simulink model "closedLoop_toTune"  (R2019a)
settings: Solver=ode14x  StartTime=0.0  StopTime=20  FixedStep=ts  RelTol=1e-3
PreLoadFcn:
  | h = 0.005;
  | k = 0.5;
PostLoadFcn:
  | controlParameters;
undefined symbols (not defined in the file): sigbuilder_block, ts
libraries: simulink x12, controlLibrary x12, mechLibrary x1
CloseFcn:
  | try,close(h1_elec_motor_brushless_dc),end
  | clear h1_elec_motor_brushless_dc
  | 
  | clear simlog_elec_motor_brushless_dc
  | clear logsout_elec_motor_brushless_dc
  | 
  | 
  | clear tout
Description:
  | Position feedback control, with servomotors, of a robot arm. Controllers are discretised.
  | 
  | Copyright 2008-2019 The MathWorks, Inc.
settings Model: DataDictionary=robotDataDictionary.sldd  EnableAccessToBaseWorkspace=off  Creator=MathWorks  LastModifiedBy=falderis
settings ConfigSet: Description=Configuration set for closed loop system
settings SolverCC: ExtrapolationOrder=1  SolverJacobianMethodControl=SparsePerturbation  AutoInsertRateTranBlk=on
settings DataIOCC: SaveFormat=StructureWithTime  SaveOutput=off  ReturnWorkspaceOutputsName=simulationOutput
settings OptimizationCC: BlockReduction=off  OptimizeBlockIOStorage=off  BufferReuse=off  GlobalBufferReuse=off  ExpressionFolding=off  LocalBlockOutputs=off  OptimizeDataStoreBuffers=off  BusAssignmentInplaceUpdate=off
settings DebuggingCC: BusObjectLabelMismatch=none  SFUnexpectedBacktrackingDiag=warning  SFNoUnconditionalDefaultTransitionDiag=warning  SFExecutionAtInitializationDiag=none  ArithmeticOperatorsInVariantConditions=warning
settings HardwareCC: ProdBitPerPointer=32  ProdBitPerSizeT=32  ProdBitPerPtrDiffT=32  ProdLargestAtomicFloat=None  ProdWordSize=32  ProdLongLongMode=on  ProdHWDeviceType=Generic->32-bit x86 compatible
settings ModelReferenceCC: ModelReferenceNumInstancesAllowed=Single  PropagateSignalLabelsOutOfModel=off
settings SFSimCC: SimUseLocalCustomCode=off
settings RTWCC: SystemTargetFile=slrt.tlc  TemplateMakefile=slrt_default_tmf  Description=Simulink Real-Time  RTWVerbose=off  RTWUseLocalCustomCode=off  CodeExecutionProfiling=on  RTWCompilerOptimization=on
settings CodeAppCC: StateflowObjectComments=on
settings SimulinkRealTimeCC: SupportVariableSizeSignals=on  PreserveStateflowLocalDataDimensions=off  RL32LogBufSizeModifier=10000000  xPCConcurrentTasks=on
settings ConfigComp: CovMetricSettings=dw  CovHtmlReporting=on  CovSaveCumulativeToWorkspaceVar=on  CovSaveSingleToWorkspaceVar=on  CovExternalEMLEnable=off  CovSFcnEnable=off
settings SimscapeCC: SimscapeNormalizeSystem=off  SimscapeLogName=mechPlant_simlog  SimscapeLogLimitData=off
settings ConfigurationSet: Description=SimMechanics 2G
settings ExplorerConfigSet: InternalSimMechanicsExplorerSettings="<ExplorerConfiguration><canonicalview>planar_xy</canonicalview><AnimationSetting><BasePlaybackSpeed>1.0</BasePlaybackSpeed><PlaybackSpeedFactor>0.5</PlaybackSpeedFactor></AnimationSetting><TilePanel><TileInfo><Tiles Columns=\"1\" Count=\"1\" Rows=\"1\"><Column Weight=\"1\"/><Row Weight=\"1\"/><Tile Height=\"1\" Width=\"1\" X=\"0\" Y=\"0\"/></Tiles></TileInfo><SceneInfo><SceneViewer><BGColor><R>1</R><G>1</G><B>1</B></BGColor><Camera><DoPerspective>off</DoPerspective><Position><X>0.403135839827215292</X><Y>0.401665542364257</Y><Z>0.341712609240549303</Z></Position><Center><X>0.0802051411090622807</X><Y>0.078734843646070099</Y><Z>0.0187819105223669576</Z></Center><Up><X>-0.408248290463863073</X><Y>0.816496580927726145</Y><Z>-0.408248290463863073</Z></Up><ViewLimDist>1</ViewLimDist><YLim>0.277558730438193679</YLim><XLim>0.533545538821605492</XLim></Camera></SceneViewer></SceneInfo></TilePanel><MechEditorPanel><Cameras/><GfxPanelCameraMap/><VideoCreator><PlaybackSpeedRatio>1.0</PlaybackSpeedRatio><FrameRate>30</FrameRate><VideoFormat>Motion JPEG AVI</VideoFormat><FrameSize>auto</FrameSize></VideoCreator></MechEditorPanel></ExplorerConfiguration>"

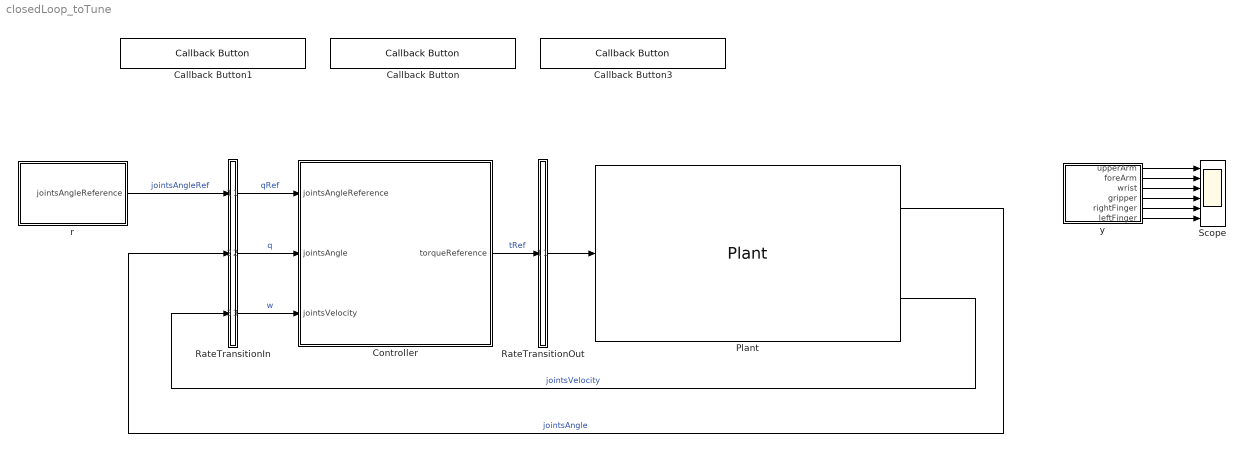
== system closedLoop_toTune ==
  Callback Button : CallbackButton  ButtonText=Open Control System Tuner
      settings: ClickFcn=|
      | h = 0.005;
      | k = 0.5;
      | controlParameters;
      | controlSystemTuner('ControlSystemTunerSession.mat')
  Callback Button1 : CallbackButton  ButtonText=Untuned Controllers
      settings: ClickFcn=|
      | h = 0.005;
      | k = 0.5;
      | controlParameters;
  Callback Button3 : CallbackButton  ButtonText=Aggressive Controller
      settings: ClickFcn=|
      | h = 1;
      | k = 1;
      | controlParameters;
  Controller : Subsystem
      mask Display: image('controller.png')
  Plant : mechLibrary/Plant  SystemSampleTime=-1
  RateTransitionIn : Subsystem
  RateTransitionOut : Subsystem
  Scope : Scope  NumInputPorts=6
  r : Subsystem
      mask Display: disp('input')
  y : Subsystem
      mask Display: disp('output')
  wires:
  Controller/1(torqueReference) -> RateTransitionOut/1(tRefIn)  "tRef"
  RateTransitionIn/1(qRef) -> Controller/1(jointsAngleReference)  "qRef"
  Plant/2 -> RateTransitionIn/3(wIn)  "jointsVelocity"
  RateTransitionOut/1(tRef) -> Plant/1
  RateTransitionIn/3(w) -> Controller/3(jointsVelocity)  "w"
  Plant/1 -> RateTransitionIn/2(qIn)  "jointsAngle"
  RateTransitionIn/2(q) -> Controller/2(jointsAngle)  "q"
  r/1(jointsAngleReference) -> RateTransitionIn/1(qRefIn)  "jointsAngleRef"
  y/1(upperArm) -> Scope/1
  y/2(foreArm) -> Scope/2
  y/3(wrist) -> Scope/3
  y/4(gripper) -> Scope/4
  y/5(rightFinger) -> Scope/5
  y/6(leftFinger) -> Scope/6

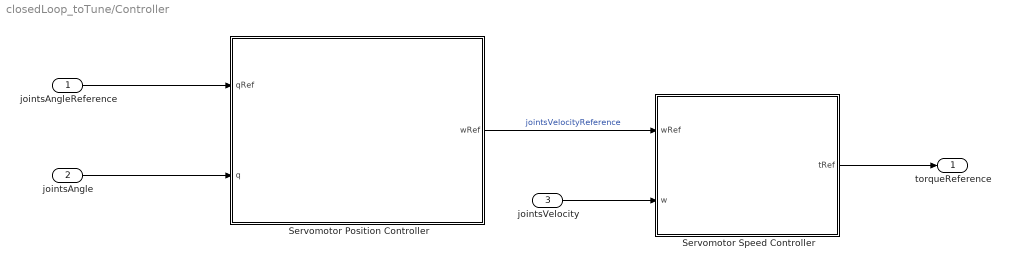
== system closedLoop_toTune/Controller ==
  jointsAngleReference : Inport  OutDataTypeStr=Bus: jointMotionBus  Unit=deg  SampleTime=ts
  jointsAngle : Inport  Port=2  OutDataTypeStr=Bus: jointMotionBus  Unit=deg  SampleTime=ts
  jointsVelocity : Inport  Port=3  OutDataTypeStr=Bus: jointVelBus  Unit=deg/s  SampleTime=ts
  Servomotor Position Controller : Subsystem  VariantControl=SV
      mask Display: image('pid.png');
  Servomotor Speed Controller : Subsystem
      mask Display: image('pi2.png');
  torqueReference : Outport  OutDataTypeStr=Bus: jointTorqueBus  Unit=N*m  SampleTime=ts
  wires:
  jointsAngle/1 -> Servomotor Position Controller/2(q)
  jointsAngleReference/1 -> Servomotor Position Controller/1(qRef)
  Servomotor Speed Controller/1(tRef) -> torqueReference/1
  Servomotor Position Controller/1(wRef) -> Servomotor Speed Controller/1(wRef)  "jointsVelocityReference"
  jointsVelocity/1 -> Servomotor Speed Controller/2(w)

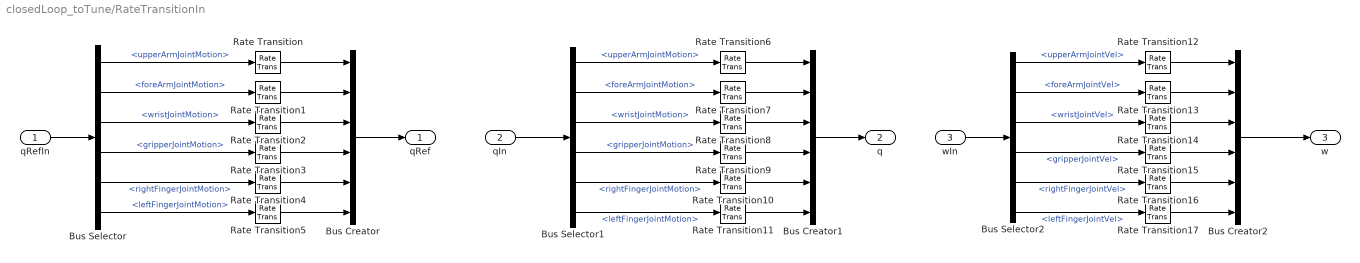
== system closedLoop_toTune/RateTransitionIn ==
  qRefIn : Inport  OutDataTypeStr=Bus: jointMotionBus  Unit=deg
  qIn : Inport  Port=2  OutDataTypeStr=Bus: jointMotionBus  Unit=deg
  wIn : Inport  Port=3  OutDataTypeStr=Bus: jointVelBus
  Bus Creator : BusCreator  Inputs=6  OutDataTypeStr=Bus: jointMotionBus
      settings: InheritFromInputs=off
  Bus Creator1 : BusCreator  Inputs=6  OutDataTypeStr=Bus: jointMotionBus
      settings: InheritFromInputs=off
  Bus Creator2 : BusCreator  Inputs=6  OutDataTypeStr=Bus: jointVelBus
      settings: InheritFromInputs=off
  Bus Selector : BusSelector  OutputSignals=upperArmJointMotion,foreArmJointMotion,wristJointMotion,gripperJointMotion,rightFingerJointMotion,leftFingerJointMotion
  Bus Selector1 : BusSelector  OutputSignals=upperArmJointMotion,foreArmJointMotion,wristJointMotion,gripperJointMotion,rightFingerJointMotion,leftFingerJointMotion
  Bus Selector2 : BusSelector  OutputSignals=upperArmJointVel,foreArmJointVel,wristJointVel,gripperJointVel,rightFingerJointVel,leftFingerJointVel
  Rate Transition{,1..17} (18 alike) : RateTransition  OutPortSampleTime=ts
  qRef : Outport  OutDataTypeStr=Bus: jointMotionBus
  q : Outport  Port=2  OutDataTypeStr=Bus: jointMotionBus
  w : Outport  Port=3  OutDataTypeStr=Bus: jointVelBus
  wires:
  Bus Selector1/6 -> Rate Transition11/1  "<leftFingerJointMotion>"
  Bus Selector1/3 -> Rate Transition8/1  "<wristJointMotion>"
  qIn/1 -> Bus Selector1/1
  Bus Selector1/1 -> Rate Transition6/1  "<upperArmJointMotion>"
  Bus Selector1/5 -> Rate Transition10/1  "<rightFingerJointMotion>"
  Bus Selector/6 -> Rate Transition5/1  "<leftFingerJointMotion>"
  Bus Selector1/4 -> Rate Transition9/1  "<gripperJointMotion>"
  Bus Selector/2 -> Rate Transition1/1  "<foreArmJointMotion>"
  Bus Selector1/2 -> Rate Transition7/1  "<foreArmJointMotion>"
  Bus Selector/3 -> Rate Transition2/1  "<wristJointMotion>"
  Bus Selector/4 -> Rate Transition3/1  "<gripperJointMotion>"
  Bus Selector/1 -> Rate Transition/1  "<upperArmJointMotion>"
  qRefIn/1 -> Bus Selector/1
  Bus Selector/5 -> Rate Transition4/1  "<rightFingerJointMotion>"
  Bus Selector2/5 -> Rate Transition16/1  "<rightFingerJointVel>"
  Bus Selector2/4 -> Rate Transition15/1  "<gripperJointVel>"
  Bus Selector2/3 -> Rate Transition14/1  "<wristJointVel>"
  wIn/1 -> Bus Selector2/1
  Bus Selector2/1 -> Rate Transition12/1  "<upperArmJointVel>"
  Bus Selector2/2 -> Rate Transition13/1  "<foreArmJointVel>"
  Bus Selector2/6 -> Rate Transition17/1  "<leftFingerJointVel>"
  Rate Transition/1 -> Bus Creator/1
  Rate Transition1/1 -> Bus Creator/2
  Rate Transition2/1 -> Bus Creator/3
  Rate Transition3/1 -> Bus Creator/4
  Rate Transition4/1 -> Bus Creator/5
  Rate Transition5/1 -> Bus Creator/6
  Bus Creator/1 -> qRef/1
  Rate Transition7/1 -> Bus Creator1/2
  Rate Transition11/1 -> Bus Creator1/6
  Bus Creator1/1 -> q/1
  Rate Transition9/1 -> Bus Creator1/4
  Rate Transition6/1 -> Bus Creator1/1
  Rate Transition8/1 -> Bus Creator1/3
  Rate Transition10/1 -> Bus Creator1/5
  Rate Transition12/1 -> Bus Creator2/1
  Rate Transition13/1 -> Bus Creator2/2
  Rate Transition14/1 -> Bus Creator2/3
  Rate Transition15/1 -> Bus Creator2/4
  Rate Transition16/1 -> Bus Creator2/5
  Rate Transition17/1 -> Bus Creator2/6
  Bus Creator2/1 -> w/1

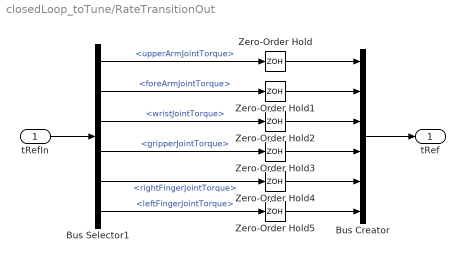
== system closedLoop_toTune/RateTransitionOut ==
  tRefIn : Inport  OutDataTypeStr=Bus: jointTorqueBus  Unit=N*m
  Bus Creator : BusCreator  Inputs=6  OutDataTypeStr=Bus: jointTorqueBus
      settings: InheritFromInputs=off
  Bus Selector1 : BusSelector  OutputSignals=upperArmJointTorque,foreArmJointTorque,wristJointTorque,gripperJointTorque,rightFingerJointTorque,leftFingerJointTorque
  Zero-Order Hold{,1..5} (6 alike) : ZeroOrderHold  SampleTime=-1
  tRef : Outport  OutDataTypeStr=Bus: jointTorqueBus  SampleTime=0
  wires:
  Bus Selector1/3 -> Zero-Order Hold2/1  "<wristJointTorque>"
  tRefIn/1 -> Bus Selector1/1
  Bus Selector1/2 -> Zero-Order Hold1/1  "<foreArmJointTorque>"
  Bus Selector1/5 -> Zero-Order Hold4/1  "<rightFingerJointTorque>"
  Bus Selector1/4 -> Zero-Order Hold3/1  "<gripperJointTorque>"
  Bus Selector1/1 -> Zero-Order Hold/1  "<upperArmJointTorque>"
  Bus Selector1/6 -> Zero-Order Hold5/1  "<leftFingerJointTorque>"
  Zero-Order Hold5/1 -> Bus Creator/6
  Zero-Order Hold4/1 -> Bus Creator/5
  Zero-Order Hold1/1 -> Bus Creator/2
  Zero-Order Hold/1 -> Bus Creator/1
  Zero-Order Hold2/1 -> Bus Creator/3
  Zero-Order Hold3/1 -> Bus Creator/4
  Bus Creator/1 -> tRef/1

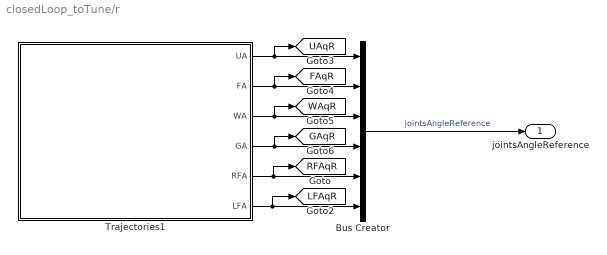
== system closedLoop_toTune/r ==
  Bus Creator : BusCreator  Inputs=6  OutDataTypeStr=Bus: jointMotionBus
      settings: InheritFromInputs=off
  Trajectories1 : Subsystem  Tag=STV Subsys  LoadFcn=sigbuilder_block('load');  StartFcn=sigbuilder_block('start');  StopFcn=sigbuilder_block('stop');  ClipboardFcn=sigbuilder_block('clipboard');  mask(Sigbuilder block){tuvar=[0:10]}
      mask help: Simulink:masks:SigbuilderBlock_MD
      mask init:
      | if ~strcmp(get_param(bdroot(gcbh),'SimulationStatus'),'stopped') tuvar = sigbuilder_block('maskInit'); end
      settings: CopyFcn=sigbuilder_block('copy');  DeleteFcn=sigbuilder_block('delete');  ModelCloseFcn=sigbuilder_block('modelClose');  PreSaveFcn=sigbuilder_block('preSave');  PauseFcn=sigbuilder_block('pause');  ContinueFcn=sigbuilder_block('continue');  NameChangeFcn=sigbuilder_block('namechange');  OpenFcn=sigbuilder_block('open',[0 30 1440 722.25 ]);  CloseFcn=sigbuilder_block('close');
      mask Display: plot(0, 0, 100, 100,[2, 2, 32, 32, 2], [68, 8, 8, 68, 68],[32, 2], [38, 38], [32, 19, 2],[53, 60, 44], [32, 17, 17, 2],[16, 16, 31, 31]);txt = getActiveGroup(gcbh);text(2, 100, txt,'verticalAlignment', 'top');
  jointsAngleReference : Outport
  tag scope: FAqR=global, GAqR=global, LFAqR=global, RFAqR=global, UAqR=global, WAqR=global
  wires:
  Trajectories1/6(LFA) -> Bus Creator/6, [LFAqR]
  Trajectories1/2(FA) -> Bus Creator/2, [FAqR]
  Trajectories1/5(RFA) -> Bus Creator/5, [RFAqR]
  Trajectories1/1(UA) -> [UAqR], Bus Creator/1
  Trajectories1/4(GA) -> [GAqR], Bus Creator/4
  Trajectories1/3(WA) -> [WAqR], Bus Creator/3
  Bus Creator/1 -> jointsAngleReference/1  "jointsAngleReference"

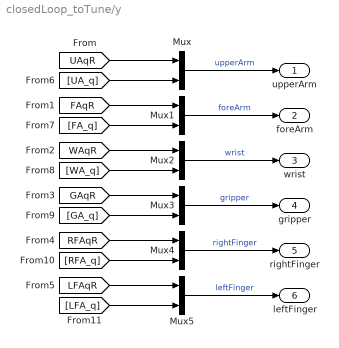
== system closedLoop_toTune/y ==
  Mux{,1..5} (6 alike) : Mux  Inputs=2
  upperArm : Outport
  foreArm : Outport  Port=2
  wrist : Outport  Port=3
  gripper : Outport  Port=4
  rightFinger : Outport  Port=5
  leftFinger : Outport  Port=6
  wires:
  Mux5/1 -> leftFinger/1  "leftFinger"
  [UA_q] -> Mux/2
  [RFA_q] -> Mux4/2
  [RFAqR] -> Mux4/1
  [UAqR] -> Mux/1
  [FAqR] -> Mux1/1
  [WAqR] -> Mux2/1
  [WA_q] -> Mux2/2
  [FA_q] -> Mux1/2
  [LFAqR] -> Mux5/1
  [LFA_q] -> Mux5/2
  [GAqR] -> Mux3/1
  [GA_q] -> Mux3/2
  Mux/1 -> upperArm/1  "upperArm"
  Mux1/1 -> foreArm/1  "foreArm"
  Mux2/1 -> wrist/1  "wrist"
  Mux4/1 -> rightFinger/1  "rightFinger"
  Mux3/1 -> gripper/1  "gripper"

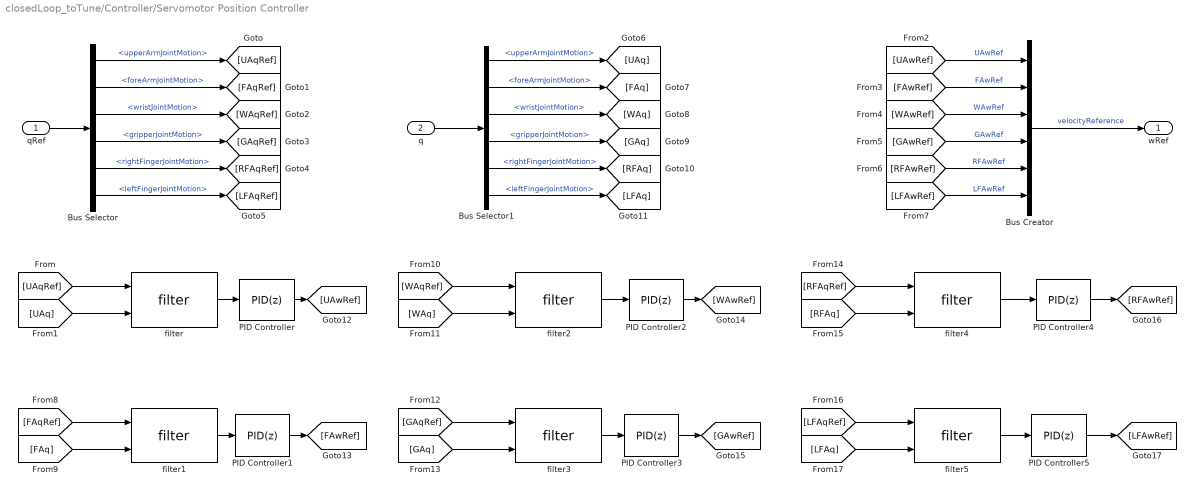
== system closedLoop_toTune/Controller/Servomotor Position Controller ==
  qRef : Inport  OutDataTypeStr=Bus: jointMotionBus  Unit=deg
  q : Inport  Port=2  OutDataTypeStr=Bus: jointMotionBus  Unit=deg
  Bus Creator : BusCreator  Inputs=6  OutDataTypeStr=Bus: jointVelBus
      settings: InheritFromInputs=off
  Bus Selector : BusSelector  OutputSignals=upperArmJointMotion,foreArmJointMotion,wristJointMotion,gripperJointMotion,rightFingerJointMotion,leftFingerJointMotion
  Bus Selector1 : BusSelector  OutputSignals=upperArmJointMotion,foreArmJointMotion,wristJointMotion,gripperJointMotion,rightFingerJointMotion,leftFingerJointMotion
  PID Controller : simulink/Continuous/PID Controller  Controller=PID  Form=Parallel  TimeDomain=Discrete-time  SampleTime=ts  IntegratorMethod=Forward Euler  FilterMethod=Forward Euler  ControllerParametersSource=internal  P=0.58  I=4.83  D=0.0027  UseFilter=on  N=0.95  TunerSelectOption=Transfer Function Based (PID Tuner App)  InitialConditionSource=internal  InitialConditionForIntegrator=0  InitialConditionForFilter=0  DifferentiatorICPrevScaledInput=0  ExternalReset=none  TrackingMode=off  Kt=1  LimitOutput=off  UpperSaturationLimit=inf  LowerSaturationLimit=-inf  LinearizeAsGain=on  AntiWindupMode=none  Kb=1  POutMin=[]  POutMax=[]  IOutMin=[]  IOutMax=[]  DOutMin=[]  DOutMax=[]  NOutMin=[]  NOutMax=[]  SumOutMin=[]  SumOutMax=[]  SaturationOutMin=[]  SaturationOutMax=[]  PParamMin=[]  PParamMax=[]  IParamMin=[]  IParamMax=[]  DParamMin=[]  DParamMax=[]  NParamMin=[]  NParamMax=[]  KbParamMin=[]  KbParamMax=[]  KtParamMin=[]  KtParamMax=[]  KbOutMin=[]  KbOutMax=[]  KtOutMin=[]  KtOutMax=[]  IntegratorOutMin=[]  IntegratorOutMax=[]  FilterOutMin=[]  FilterOutMax=[]  SumI1OutMin=[]  SumI1OutMax=[]  SumI2OutMin=[]  SumI2OutMax=[]  SumI3OutMin=[]  SumI3OutMax=[]  SumI4OutMin=[]  SumI4OutMax=[]  SumDOutMin=[]  SumDOutMax=[]  DifferentiatorOutMin=[]  DifferentiatorOutMax=[]  FilterDiffOutCoefMin=[]  FilterDiffOutCoefMax=[]  ReciprocalOutMin=[]  ReciprocalOutMax=[]  SumDenOutMin=[]  SumDenOutMax=[]  SumNumOutMin=[]  SumNumOutMax=[]  DivideOutMin=[]  DivideOutMax=[]  IntegratorContinuousStateAttributes=''  IntegratorStateMustResolveToSignalObject=off  IntegratorRTWStateStorageClass=Auto  FilterContinuousStateAttributes=''  FilterStateMustResolveToSignalObject=off  FilterRTWStateStorageClass=Auto  ParallelPVariant=InternalParameters  IdealPVariant=Disabled  IVariant=InternalParameters  DVariant=InternalParameters  IntegratorVariant=Discrete  SatVariant=Disabled  AWVariant=Passthrough  PCopyVariant=Disabled  TRVariant=Disabled  FdbkBlocksVariant=Forward  IdealPFdbkVariant=Disabled  SatFdbkVariant=Disabled  DerivativeFilterVariant=ForwardEulerFilter  NVariant=InternalParameters  NCopyVariant=Disabled  FilterICVariant=InternalICsFilter  IntegratorICVariant=InternalICs  ExternalResetVariant=Disabled  TRSumVariant=Passthrough  SumFdbkVariant=Disabled  SumVariant=Sum_PID
  PID Controller1 : simulink/Continuous/PID Controller  Controller=PID  Form=Parallel  TimeDomain=Discrete-time  SampleTime=ts  IntegratorMethod=Forward Euler  FilterMethod=Forward Euler  ControllerParametersSource=internal  P=0.11915  I=0.918  D=0.00315  UseFilter=on  N=1.15  TunerSelectOption=Transfer Function Based (PID Tuner App)  InitialConditionSource=internal  InitialConditionForIntegrator=0  InitialConditionForFilter=0  DifferentiatorICPrevScaledInput=0  ExternalReset=none  TrackingMode=off  Kt=1  LimitOutput=off  UpperSaturationLimit=inf  LowerSaturationLimit=-inf  LinearizeAsGain=on  AntiWindupMode=none  Kb=1  POutMin=[]  POutMax=[]  IOutMin=[]  IOutMax=[]  DOutMin=[]  DOutMax=[]  NOutMin=[]  NOutMax=[]  SumOutMin=[]  SumOutMax=[]  SaturationOutMin=[]  SaturationOutMax=[]  PParamMin=[]  PParamMax=[]  IParamMin=[]  IParamMax=[]  DParamMin=[]  DParamMax=[]  NParamMin=[]  NParamMax=[]  KbParamMin=[]  KbParamMax=[]  KtParamMin=[]  KtParamMax=[]  KbOutMin=[]  KbOutMax=[]  KtOutMin=[]  KtOutMax=[]  IntegratorOutMin=[]  IntegratorOutMax=[]  FilterOutMin=[]  FilterOutMax=[]  SumI1OutMin=[]  SumI1OutMax=[]  SumI2OutMin=[]  SumI2OutMax=[]  SumI3OutMin=[]  SumI3OutMax=[]  SumI4OutMin=[]  SumI4OutMax=[]  SumDOutMin=[]  SumDOutMax=[]  DifferentiatorOutMin=[]  DifferentiatorOutMax=[]  FilterDiffOutCoefMin=[]  FilterDiffOutCoefMax=[]  ReciprocalOutMin=[]  ReciprocalOutMax=[]  SumDenOutMin=[]  SumDenOutMax=[]  SumNumOutMin=[]  SumNumOutMax=[]  DivideOutMin=[]  DivideOutMax=[]  IntegratorContinuousStateAttributes=''  IntegratorStateMustResolveToSignalObject=off  IntegratorRTWStateStorageClass=Auto  FilterContinuousStateAttributes=''  FilterStateMustResolveToSignalObject=off  FilterRTWStateStorageClass=Auto  ParallelPVariant=InternalParameters  IdealPVariant=Disabled  IVariant=InternalParameters  DVariant=InternalParameters  IntegratorVariant=Discrete  SatVariant=Disabled  AWVariant=Passthrough  PCopyVariant=Disabled  TRVariant=Disabled  FdbkBlocksVariant=Forward  IdealPFdbkVariant=Disabled  SatFdbkVariant=Disabled  DerivativeFilterVariant=ForwardEulerFilter  NVariant=InternalParameters  NCopyVariant=Disabled  FilterICVariant=InternalICsFilter  IntegratorICVariant=InternalICs  ExternalResetVariant=Disabled  TRSumVariant=Passthrough  SumFdbkVariant=Disabled  SumVariant=Sum_PID
  PID Controller2 : simulink/Continuous/PID Controller  Controller=PID  Form=Parallel  TimeDomain=Discrete-time  SampleTime=ts  IntegratorMethod=Forward Euler  FilterMethod=Forward Euler  ControllerParametersSource=internal  P=0.468  I=3.6488  D=0.0031  UseFilter=on  N=3.7035  TunerSelectOption=Transfer Function Based (PID Tuner App)  InitialConditionSource=internal  InitialConditionForIntegrator=0  InitialConditionForFilter=0  DifferentiatorICPrevScaledInput=0  ExternalReset=none  TrackingMode=off  Kt=1  LimitOutput=off  UpperSaturationLimit=inf  LowerSaturationLimit=-inf  LinearizeAsGain=on  AntiWindupMode=none  Kb=1  POutMin=[]  POutMax=[]  IOutMin=[]  IOutMax=[]  DOutMin=[]  DOutMax=[]  NOutMin=[]  NOutMax=[]  SumOutMin=[]  SumOutMax=[]  SaturationOutMin=[]  SaturationOutMax=[]  PParamMin=[]  PParamMax=[]  IParamMin=[]  IParamMax=[]  DParamMin=[]  DParamMax=[]  NParamMin=[]  NParamMax=[]  KbParamMin=[]  KbParamMax=[]  KtParamMin=[]  KtParamMax=[]  KbOutMin=[]  KbOutMax=[]  KtOutMin=[]  KtOutMax=[]  IntegratorOutMin=[]  IntegratorOutMax=[]  FilterOutMin=[]  FilterOutMax=[]  SumI1OutMin=[]  SumI1OutMax=[]  SumI2OutMin=[]  SumI2OutMax=[]  SumI3OutMin=[]  SumI3OutMax=[]  SumI4OutMin=[]  SumI4OutMax=[]  SumDOutMin=[]  SumDOutMax=[]  DifferentiatorOutMin=[]  DifferentiatorOutMax=[]  FilterDiffOutCoefMin=[]  FilterDiffOutCoefMax=[]  ReciprocalOutMin=[]  ReciprocalOutMax=[]  SumDenOutMin=[]  SumDenOutMax=[]  SumNumOutMin=[]  SumNumOutMax=[]  DivideOutMin=[]  DivideOutMax=[]  IntegratorContinuousStateAttributes=''  IntegratorStateMustResolveToSignalObject=off  IntegratorRTWStateStorageClass=Auto  FilterContinuousStateAttributes=''  FilterStateMustResolveToSignalObject=off  FilterRTWStateStorageClass=Auto  ParallelPVariant=InternalParameters  IdealPVariant=Disabled  IVariant=InternalParameters  DVariant=InternalParameters  IntegratorVariant=Discrete  SatVariant=Disabled  AWVariant=Passthrough  PCopyVariant=Disabled  TRVariant=Disabled  FdbkBlocksVariant=Forward  IdealPFdbkVariant=Disabled  SatFdbkVariant=Disabled  DerivativeFilterVariant=ForwardEulerFilter  NVariant=InternalParameters  NCopyVariant=Disabled  FilterICVariant=InternalICsFilter  IntegratorICVariant=InternalICs  ExternalResetVariant=Disabled  TRSumVariant=Passthrough  SumFdbkVariant=Disabled  SumVariant=Sum_PID
  PID Controller3 : simulink/Continuous/PID Controller  Controller=PID  Form=Parallel  TimeDomain=Discrete-time  SampleTime=ts  IntegratorMethod=Forward Euler  FilterMethod=Forward Euler  ControllerParametersSource=internal  P=0.30195  I=0.20875  D=0.00335  UseFilter=on  N=3.677  TunerSelectOption=Transfer Function Based (PID Tuner App)  InitialConditionSource=internal  InitialConditionForIntegrator=0  InitialConditionForFilter=0  DifferentiatorICPrevScaledInput=0  ExternalReset=none  TrackingMode=off  Kt=1  LimitOutput=off  UpperSaturationLimit=inf  LowerSaturationLimit=-inf  LinearizeAsGain=on  AntiWindupMode=none  Kb=1  POutMin=[]  POutMax=[]  IOutMin=[]  IOutMax=[]  DOutMin=[]  DOutMax=[]  NOutMin=[]  NOutMax=[]  SumOutMin=[]  SumOutMax=[]  SaturationOutMin=[]  SaturationOutMax=[]  PParamMin=[]  PParamMax=[]  IParamMin=[]  IParamMax=[]  DParamMin=[]  DParamMax=[]  NParamMin=[]  NParamMax=[]  KbParamMin=[]  KbParamMax=[]  KtParamMin=[]  KtParamMax=[]  KbOutMin=[]  KbOutMax=[]  KtOutMin=[]  KtOutMax=[]  IntegratorOutMin=[]  IntegratorOutMax=[]  FilterOutMin=[]  FilterOutMax=[]  SumI1OutMin=[]  SumI1OutMax=[]  SumI2OutMin=[]  SumI2OutMax=[]  SumI3OutMin=[]  SumI3OutMax=[]  SumI4OutMin=[]  SumI4OutMax=[]  SumDOutMin=[]  SumDOutMax=[]  DifferentiatorOutMin=[]  DifferentiatorOutMax=[]  FilterDiffOutCoefMin=[]  FilterDiffOutCoefMax=[]  ReciprocalOutMin=[]  ReciprocalOutMax=[]  SumDenOutMin=[]  SumDenOutMax=[]  SumNumOutMin=[]  SumNumOutMax=[]  DivideOutMin=[]  DivideOutMax=[]  IntegratorContinuousStateAttributes=''  IntegratorStateMustResolveToSignalObject=off  IntegratorRTWStateStorageClass=Auto  FilterContinuousStateAttributes=''  FilterStateMustResolveToSignalObject=off  FilterRTWStateStorageClass=Auto  ParallelPVariant=InternalParameters  IdealPVariant=Disabled  IVariant=InternalParameters  DVariant=InternalParameters  IntegratorVariant=Discrete  SatVariant=Disabled  AWVariant=Passthrough  PCopyVariant=Disabled  TRVariant=Disabled  FdbkBlocksVariant=Forward  IdealPFdbkVariant=Disabled  SatFdbkVariant=Disabled  DerivativeFilterVariant=ForwardEulerFilter  NVariant=InternalParameters  NCopyVariant=Disabled  FilterICVariant=InternalICsFilter  IntegratorICVariant=InternalICs  ExternalResetVariant=Disabled  TRSumVariant=Passthrough  SumFdbkVariant=Disabled  SumVariant=Sum_PID
  PID Controller4 : simulink/Continuous/PID Controller  Controller=PID  Form=Parallel  TimeDomain=Discrete-time  SampleTime=ts  IntegratorMethod=Forward Euler  FilterMethod=Forward Euler  ControllerParametersSource=internal  P=0.425  I=3.52  D=0.0036  UseFilter=on  N=1.2175  TunerSelectOption=Transfer Function Based (PID Tuner App)  InitialConditionSource=internal  InitialConditionForIntegrator=0  InitialConditionForFilter=0  DifferentiatorICPrevScaledInput=0  ExternalReset=none  TrackingMode=off  Kt=1  LimitOutput=off  UpperSaturationLimit=inf  LowerSaturationLimit=-inf  LinearizeAsGain=on  AntiWindupMode=none  Kb=1  POutMin=[]  POutMax=[]  IOutMin=[]  IOutMax=[]  DOutMin=[]  DOutMax=[]  NOutMin=[]  NOutMax=[]  SumOutMin=[]  SumOutMax=[]  SaturationOutMin=[]  SaturationOutMax=[]  PParamMin=[]  PParamMax=[]  IParamMin=[]  IParamMax=[]  DParamMin=[]  DParamMax=[]  NParamMin=[]  NParamMax=[]  KbParamMin=[]  KbParamMax=[]  KtParamMin=[]  KtParamMax=[]  KbOutMin=[]  KbOutMax=[]  KtOutMin=[]  KtOutMax=[]  IntegratorOutMin=[]  IntegratorOutMax=[]  FilterOutMin=[]  FilterOutMax=[]  SumI1OutMin=[]  SumI1OutMax=[]  SumI2OutMin=[]  SumI2OutMax=[]  SumI3OutMin=[]  SumI3OutMax=[]  SumI4OutMin=[]  SumI4OutMax=[]  SumDOutMin=[]  SumDOutMax=[]  DifferentiatorOutMin=[]  DifferentiatorOutMax=[]  FilterDiffOutCoefMin=[]  FilterDiffOutCoefMax=[]  ReciprocalOutMin=[]  ReciprocalOutMax=[]  SumDenOutMin=[]  SumDenOutMax=[]  SumNumOutMin=[]  SumNumOutMax=[]  DivideOutMin=[]  DivideOutMax=[]  IntegratorContinuousStateAttributes=''  IntegratorStateMustResolveToSignalObject=off  IntegratorRTWStateStorageClass=Auto  FilterContinuousStateAttributes=''  FilterStateMustResolveToSignalObject=off  FilterRTWStateStorageClass=Auto  ParallelPVariant=InternalParameters  IdealPVariant=Disabled  IVariant=InternalParameters  DVariant=InternalParameters  IntegratorVariant=Discrete  SatVariant=Disabled  AWVariant=Passthrough  PCopyVariant=Disabled  TRVariant=Disabled  FdbkBlocksVariant=Forward  IdealPFdbkVariant=Disabled  SatFdbkVariant=Disabled  DerivativeFilterVariant=ForwardEulerFilter  NVariant=InternalParameters  NCopyVariant=Disabled  FilterICVariant=InternalICsFilter  IntegratorICVariant=InternalICs  ExternalResetVariant=Disabled  TRSumVariant=Passthrough  SumFdbkVariant=Disabled  SumVariant=Sum_PID
  PID Controller5 : simulink/Continuous/PID Controller  Controller=PID  Form=Parallel  TimeDomain=Discrete-time  SampleTime=ts  IntegratorMethod=Forward Euler  FilterMethod=Forward Euler  ControllerParametersSource=internal  P=0.58  I=4.83  D=0.0027  UseFilter=on  N=0.95  TunerSelectOption=Transfer Function Based (PID Tuner App)  InitialConditionSource=internal  InitialConditionForIntegrator=0  InitialConditionForFilter=0  DifferentiatorICPrevScaledInput=0  ExternalReset=none  TrackingMode=off  Kt=1  LimitOutput=off  UpperSaturationLimit=inf  LowerSaturationLimit=-inf  LinearizeAsGain=on  AntiWindupMode=none  Kb=1  POutMin=[]  POutMax=[]  IOutMin=[]  IOutMax=[]  DOutMin=[]  DOutMax=[]  NOutMin=[]  NOutMax=[]  SumOutMin=[]  SumOutMax=[]  SaturationOutMin=[]  SaturationOutMax=[]  PParamMin=[]  PParamMax=[]  IParamMin=[]  IParamMax=[]  DParamMin=[]  DParamMax=[]  NParamMin=[]  NParamMax=[]  KbParamMin=[]  KbParamMax=[]  KtParamMin=[]  KtParamMax=[]  KbOutMin=[]  KbOutMax=[]  KtOutMin=[]  KtOutMax=[]  IntegratorOutMin=[]  IntegratorOutMax=[]  FilterOutMin=[]  FilterOutMax=[]  SumI1OutMin=[]  SumI1OutMax=[]  SumI2OutMin=[]  SumI2OutMax=[]  SumI3OutMin=[]  SumI3OutMax=[]  SumI4OutMin=[]  SumI4OutMax=[]  SumDOutMin=[]  SumDOutMax=[]  DifferentiatorOutMin=[]  DifferentiatorOutMax=[]  FilterDiffOutCoefMin=[]  FilterDiffOutCoefMax=[]  ReciprocalOutMin=[]  ReciprocalOutMax=[]  SumDenOutMin=[]  SumDenOutMax=[]  SumNumOutMin=[]  SumNumOutMax=[]  DivideOutMin=[]  DivideOutMax=[]  IntegratorContinuousStateAttributes=''  IntegratorStateMustResolveToSignalObject=off  IntegratorRTWStateStorageClass=Auto  FilterContinuousStateAttributes=''  FilterStateMustResolveToSignalObject=off  FilterRTWStateStorageClass=Auto  ParallelPVariant=InternalParameters  IdealPVariant=Disabled  IVariant=InternalParameters  DVariant=InternalParameters  IntegratorVariant=Discrete  SatVariant=Disabled  AWVariant=Passthrough  PCopyVariant=Disabled  TRVariant=Disabled  FdbkBlocksVariant=Forward  IdealPFdbkVariant=Disabled  SatFdbkVariant=Disabled  DerivativeFilterVariant=ForwardEulerFilter  NVariant=InternalParameters  NCopyVariant=Disabled  FilterICVariant=InternalICsFilter  IntegratorICVariant=InternalICs  ExternalResetVariant=Disabled  TRSumVariant=Passthrough  SumFdbkVariant=Disabled  SumVariant=Sum_PID
  filter{,1..5} (6 alike) : controlLibrary/filter  tc=1e-2  sampleTime=ts
  wRef : Outport  OutDataTypeStr=Bus: jointVelBus  Unit=deg/s
  wires:
  qRef/1 -> Bus Selector/1
  q/1 -> Bus Selector1/1
  Bus Selector/1 -> [UAqRef]  "<upperArmJointMotion>"
  Bus Selector/2 -> [FAqRef]  "<foreArmJointMotion>"
  Bus Selector/3 -> [WAqRef]  "<wristJointMotion>"
  Bus Selector/4 -> [GAqRef]  "<gripperJointMotion>"
  Bus Selector/5 -> [RFAqRef]  "<rightFingerJointMotion>"
  Bus Selector/6 -> [LFAqRef]  "<leftFingerJointMotion>"
  Bus Selector1/1 -> [UAq]  "<upperArmJointMotion>"
  Bus Selector1/3 -> [WAq]  "<wristJointMotion>"
  Bus Selector1/2 -> [FAq]  "<foreArmJointMotion>"
  Bus Selector1/5 -> [RFAq]  "<rightFingerJointMotion>"
  Bus Selector1/4 -> [GAq]  "<gripperJointMotion>"
  Bus Selector1/6 -> [LFAq]  "<leftFingerJointMotion>"
  [UAwRef] -> Bus Creator/1  "UAwRef"
  [FAwRef] -> Bus Creator/2  "FAwRef"
  [WAwRef] -> Bus Creator/3  "WAwRef"
  [GAwRef] -> Bus Creator/4  "GAwRef"
  [RFAwRef] -> Bus Creator/5  "RFAwRef"
  [LFAwRef] -> Bus Creator/6  "LFAwRef"
  Bus Creator/1 -> wRef/1  "velocityReference"
  filter5/1 -> PID Controller5/1
  [RFAq] -> filter4/2
  [LFAq] -> filter5/2
  [FAqRef] -> filter1/1
  [GAqRef] -> filter3/1
  filter3/1 -> PID Controller3/1
  [UAq] -> filter/2
  [RFAqRef] -> filter4/1
  [WAq] -> filter2/2
  [UAqRef] -> filter/1
  filter2/1 -> PID Controller2/1
  [WAqRef] -> filter2/1
  [FAq] -> filter1/2
  [GAq] -> filter3/2
  [LFAqRef] -> filter5/1
  filter4/1 -> PID Controller4/1
  filter/1 -> PID Controller/1
  PID Controller/1 -> [UAwRef]
  PID Controller2/1 -> [WAwRef]
  PID Controller3/1 -> [GAwRef]
  PID Controller4/1 -> [RFAwRef]
  PID Controller5/1 -> [LFAwRef]
  filter1/1 -> PID Controller1/1
  PID Controller1/1 -> [FAwRef]

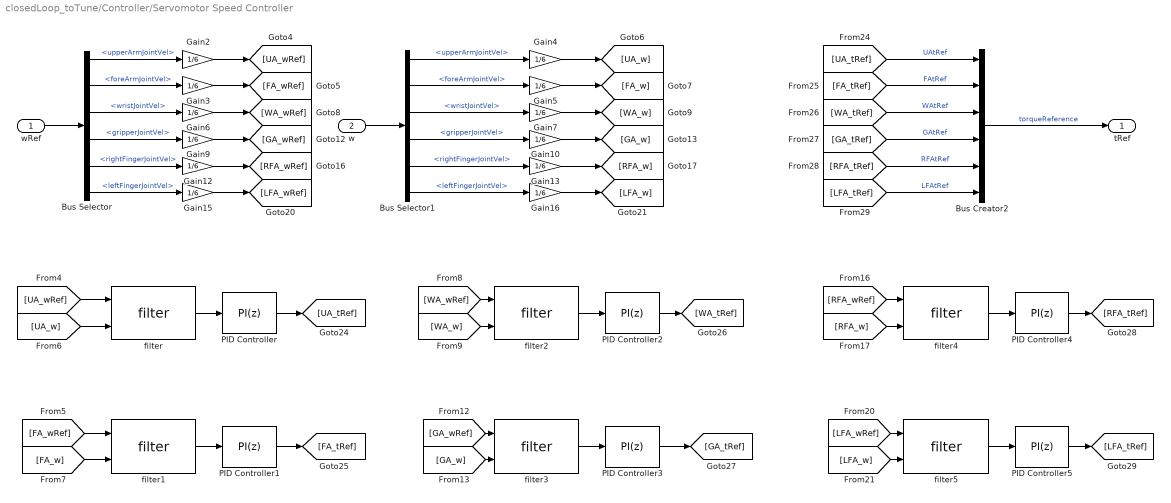
== system closedLoop_toTune/Controller/Servomotor Speed Controller ==
  wRef : Inport  OutDataTypeStr=Bus: jointVelBus
  w : Inport  Port=2  OutDataTypeStr=Bus: jointVelBus
  Bus Creator2 : BusCreator  Inputs=6  OutDataTypeStr=Bus: jointTorqueBus
      settings: InheritFromInputs=off
  Bus Selector : BusSelector  OutputSignals=upperArmJointVel,foreArmJointVel,wristJointVel,gripperJointVel,rightFingerJointVel,leftFingerJointVel
  Bus Selector1 : BusSelector  OutputSignals=upperArmJointVel,foreArmJointVel,wristJointVel,gripperJointVel,rightFingerJointVel,leftFingerJointVel
  Gain{2..7,9..10,12..13,15..16} (12 alike) : Gain  Gain=1/6
  PID Controller : simulink/Continuous/PID Controller  Controller=PI  Form=Parallel  TimeDomain=Discrete-time  SampleTime=ts  IntegratorMethod=Forward Euler  FilterMethod=Forward Euler  ControllerParametersSource=internal  P=0.04  I=0.875  D=0  UseFilter=on  N=0  TunerSelectOption=Transfer Function Based (PID Tuner App)  InitialConditionSource=internal  InitialConditionForIntegrator=0  InitialConditionForFilter=0  DifferentiatorICPrevScaledInput=0  ExternalReset=none  TrackingMode=off  Kt=1  LimitOutput=off  UpperSaturationLimit=inf  LowerSaturationLimit=-inf  LinearizeAsGain=on  AntiWindupMode=none  Kb=1  POutMin=[]  POutMax=[]  IOutMin=[]  IOutMax=[]  DOutMin=[]  DOutMax=[]  NOutMin=[]  NOutMax=[]  SumOutMin=[]  SumOutMax=[]  SaturationOutMin=[]  SaturationOutMax=[]  PParamMin=[]  PParamMax=[]  IParamMin=[]  IParamMax=[]  DParamMin=[]  DParamMax=[]  NParamMin=[]  NParamMax=[]  KbParamMin=[]  KbParamMax=[]  KtParamMin=[]  KtParamMax=[]  KbOutMin=[]  KbOutMax=[]  KtOutMin=[]  KtOutMax=[]  IntegratorOutMin=[]  IntegratorOutMax=[]  FilterOutMin=[]  FilterOutMax=[]  SumI1OutMin=[]  SumI1OutMax=[]  SumI2OutMin=[]  SumI2OutMax=[]  SumI3OutMin=[]  SumI3OutMax=[]  SumI4OutMin=[]  SumI4OutMax=[]  SumDOutMin=[]  SumDOutMax=[]  DifferentiatorOutMin=[]  DifferentiatorOutMax=[]  FilterDiffOutCoefMin=[]  FilterDiffOutCoefMax=[]  ReciprocalOutMin=[]  ReciprocalOutMax=[]  SumDenOutMin=[]  SumDenOutMax=[]  SumNumOutMin=[]  SumNumOutMax=[]  DivideOutMin=[]  DivideOutMax=[]  IntegratorContinuousStateAttributes=''  IntegratorStateMustResolveToSignalObject=off  IntegratorRTWStateStorageClass=Auto  FilterContinuousStateAttributes=''  FilterStateMustResolveToSignalObject=off  FilterRTWStateStorageClass=Auto  ParallelPVariant=InternalParameters  IdealPVariant=Disabled  IVariant=InternalParameters  DVariant=Disabled  IntegratorVariant=Discrete  SatVariant=Disabled  AWVariant=Passthrough  PCopyVariant=Disabled  TRVariant=Disabled  FdbkBlocksVariant=Forward  IdealPFdbkVariant=Disabled  SatFdbkVariant=Disabled  DerivativeFilterVariant=Disabled  NVariant=Disabled  NCopyVariant=Disabled_SignalSpec  FilterICVariant=Disabled  IntegratorICVariant=InternalICs  ExternalResetVariant=Disabled  TRSumVariant=Passthrough  SumFdbkVariant=Disabled  SumVariant=Sum_PI
  PID Controller1 : simulink/Continuous/PID Controller  Controller=PI  Form=Parallel  TimeDomain=Discrete-time  SampleTime=ts  IntegratorMethod=Forward Euler  FilterMethod=Forward Euler  ControllerParametersSource=internal  P=0.0038  I=0.046  D=0  UseFilter=on  N=0  TunerSelectOption=Transfer Function Based (PID Tuner App)  InitialConditionSource=internal  InitialConditionForIntegrator=0  InitialConditionForFilter=0  DifferentiatorICPrevScaledInput=0  ExternalReset=none  TrackingMode=off  Kt=1  LimitOutput=off  UpperSaturationLimit=inf  LowerSaturationLimit=-inf  LinearizeAsGain=on  AntiWindupMode=none  Kb=1  POutMin=[]  POutMax=[]  IOutMin=[]  IOutMax=[]  DOutMin=[]  DOutMax=[]  NOutMin=[]  NOutMax=[]  SumOutMin=[]  SumOutMax=[]  SaturationOutMin=[]  SaturationOutMax=[]  PParamMin=[]  PParamMax=[]  IParamMin=[]  IParamMax=[]  DParamMin=[]  DParamMax=[]  NParamMin=[]  NParamMax=[]  KbParamMin=[]  KbParamMax=[]  KtParamMin=[]  KtParamMax=[]  KbOutMin=[]  KbOutMax=[]  KtOutMin=[]  KtOutMax=[]  IntegratorOutMin=[]  IntegratorOutMax=[]  FilterOutMin=[]  FilterOutMax=[]  SumI1OutMin=[]  SumI1OutMax=[]  SumI2OutMin=[]  SumI2OutMax=[]  SumI3OutMin=[]  SumI3OutMax=[]  SumI4OutMin=[]  SumI4OutMax=[]  SumDOutMin=[]  SumDOutMax=[]  DifferentiatorOutMin=[]  DifferentiatorOutMax=[]  FilterDiffOutCoefMin=[]  FilterDiffOutCoefMax=[]  ReciprocalOutMin=[]  ReciprocalOutMax=[]  SumDenOutMin=[]  SumDenOutMax=[]  SumNumOutMin=[]  SumNumOutMax=[]  DivideOutMin=[]  DivideOutMax=[]  IntegratorContinuousStateAttributes=''  IntegratorStateMustResolveToSignalObject=off  IntegratorRTWStateStorageClass=Auto  FilterContinuousStateAttributes=''  FilterStateMustResolveToSignalObject=off  FilterRTWStateStorageClass=Auto  ParallelPVariant=InternalParameters  IdealPVariant=Disabled  IVariant=InternalParameters  DVariant=Disabled  IntegratorVariant=Discrete  SatVariant=Disabled  AWVariant=Passthrough  PCopyVariant=Disabled  TRVariant=Disabled  FdbkBlocksVariant=Forward  IdealPFdbkVariant=Disabled  SatFdbkVariant=Disabled  DerivativeFilterVariant=Disabled  NVariant=Disabled  NCopyVariant=Disabled_SignalSpec  FilterICVariant=Disabled  IntegratorICVariant=InternalICs  ExternalResetVariant=Disabled  TRSumVariant=Passthrough  SumFdbkVariant=Disabled  SumVariant=Sum_PI
  PID Controller2 : simulink/Continuous/PID Controller  Controller=PI  Form=Parallel  TimeDomain=Discrete-time  SampleTime=ts  IntegratorMethod=Forward Euler  FilterMethod=Forward Euler  ControllerParametersSource=internal  P=0.01  I=0.035  D=0  UseFilter=on  N=0  TunerSelectOption=Transfer Function Based (PID Tuner App)  InitialConditionSource=internal  InitialConditionForIntegrator=0  InitialConditionForFilter=0  DifferentiatorICPrevScaledInput=0  ExternalReset=none  TrackingMode=off  Kt=1  LimitOutput=off  UpperSaturationLimit=inf  LowerSaturationLimit=-inf  LinearizeAsGain=on  AntiWindupMode=none  Kb=1  POutMin=[]  POutMax=[]  IOutMin=[]  IOutMax=[]  DOutMin=[]  DOutMax=[]  NOutMin=[]  NOutMax=[]  SumOutMin=[]  SumOutMax=[]  SaturationOutMin=[]  SaturationOutMax=[]  PParamMin=[]  PParamMax=[]  IParamMin=[]  IParamMax=[]  DParamMin=[]  DParamMax=[]  NParamMin=[]  NParamMax=[]  KbParamMin=[]  KbParamMax=[]  KtParamMin=[]  KtParamMax=[]  KbOutMin=[]  KbOutMax=[]  KtOutMin=[]  KtOutMax=[]  IntegratorOutMin=[]  IntegratorOutMax=[]  FilterOutMin=[]  FilterOutMax=[]  SumI1OutMin=[]  SumI1OutMax=[]  SumI2OutMin=[]  SumI2OutMax=[]  SumI3OutMin=[]  SumI3OutMax=[]  SumI4OutMin=[]  SumI4OutMax=[]  SumDOutMin=[]  SumDOutMax=[]  DifferentiatorOutMin=[]  DifferentiatorOutMax=[]  FilterDiffOutCoefMin=[]  FilterDiffOutCoefMax=[]  ReciprocalOutMin=[]  ReciprocalOutMax=[]  SumDenOutMin=[]  SumDenOutMax=[]  SumNumOutMin=[]  SumNumOutMax=[]  DivideOutMin=[]  DivideOutMax=[]  IntegratorContinuousStateAttributes=''  IntegratorStateMustResolveToSignalObject=off  IntegratorRTWStateStorageClass=Auto  FilterContinuousStateAttributes=''  FilterStateMustResolveToSignalObject=off  FilterRTWStateStorageClass=Auto  ParallelPVariant=InternalParameters  IdealPVariant=Disabled  IVariant=InternalParameters  DVariant=Disabled  IntegratorVariant=Discrete  SatVariant=Disabled  AWVariant=Passthrough  PCopyVariant=Disabled  TRVariant=Disabled  FdbkBlocksVariant=Forward  IdealPFdbkVariant=Disabled  SatFdbkVariant=Disabled  DerivativeFilterVariant=Disabled  NVariant=Disabled  NCopyVariant=Disabled_SignalSpec  FilterICVariant=Disabled  IntegratorICVariant=InternalICs  ExternalResetVariant=Disabled  TRSumVariant=Passthrough  SumFdbkVariant=Disabled  SumVariant=Sum_PI
  PID Controller3 : simulink/Continuous/PID Controller  Controller=PI  Form=Parallel  TimeDomain=Discrete-time  SampleTime=ts  IntegratorMethod=Forward Euler  FilterMethod=Forward Euler  ControllerParametersSource=internal  P=0.001  I=0.02  D=0  UseFilter=on  N=0  TunerSelectOption=Transfer Function Based (PID Tuner App)  InitialConditionSource=internal  InitialConditionForIntegrator=0  InitialConditionForFilter=0  DifferentiatorICPrevScaledInput=0  ExternalReset=none  TrackingMode=off  Kt=1  LimitOutput=off  UpperSaturationLimit=inf  LowerSaturationLimit=-inf  LinearizeAsGain=on  AntiWindupMode=none  Kb=1  POutMin=[]  POutMax=[]  IOutMin=[]  IOutMax=[]  DOutMin=[]  DOutMax=[]  NOutMin=[]  NOutMax=[]  SumOutMin=[]  SumOutMax=[]  SaturationOutMin=[]  SaturationOutMax=[]  PParamMin=[]  PParamMax=[]  IParamMin=[]  IParamMax=[]  DParamMin=[]  DParamMax=[]  NParamMin=[]  NParamMax=[]  KbParamMin=[]  KbParamMax=[]  KtParamMin=[]  KtParamMax=[]  KbOutMin=[]  KbOutMax=[]  KtOutMin=[]  KtOutMax=[]  IntegratorOutMin=[]  IntegratorOutMax=[]  FilterOutMin=[]  FilterOutMax=[]  SumI1OutMin=[]  SumI1OutMax=[]  SumI2OutMin=[]  SumI2OutMax=[]  SumI3OutMin=[]  SumI3OutMax=[]  SumI4OutMin=[]  SumI4OutMax=[]  SumDOutMin=[]  SumDOutMax=[]  DifferentiatorOutMin=[]  DifferentiatorOutMax=[]  FilterDiffOutCoefMin=[]  FilterDiffOutCoefMax=[]  ReciprocalOutMin=[]  ReciprocalOutMax=[]  SumDenOutMin=[]  SumDenOutMax=[]  SumNumOutMin=[]  SumNumOutMax=[]  DivideOutMin=[]  DivideOutMax=[]  IntegratorContinuousStateAttributes=''  IntegratorStateMustResolveToSignalObject=off  IntegratorRTWStateStorageClass=Auto  FilterContinuousStateAttributes=''  FilterStateMustResolveToSignalObject=off  FilterRTWStateStorageClass=Auto  ParallelPVariant=InternalParameters  IdealPVariant=Disabled  IVariant=InternalParameters  DVariant=Disabled  IntegratorVariant=Discrete  SatVariant=Disabled  AWVariant=Passthrough  PCopyVariant=Disabled  TRVariant=Disabled  FdbkBlocksVariant=Forward  IdealPFdbkVariant=Disabled  SatFdbkVariant=Disabled  DerivativeFilterVariant=Disabled  NVariant=Disabled  NCopyVariant=Disabled_SignalSpec  FilterICVariant=Disabled  IntegratorICVariant=InternalICs  ExternalResetVariant=Disabled  TRSumVariant=Passthrough  SumFdbkVariant=Disabled  SumVariant=Sum_PI
  PID Controller4 : simulink/Continuous/PID Controller  Controller=PI  Form=Parallel  TimeDomain=Discrete-time  SampleTime=ts  IntegratorMethod=Forward Euler  FilterMethod=Forward Euler  ControllerParametersSource=internal  P=0.00225  I=0.015  D=0  UseFilter=on  N=0  TunerSelectOption=Transfer Function Based (PID Tuner App)  InitialConditionSource=internal  InitialConditionForIntegrator=0  InitialConditionForFilter=0  DifferentiatorICPrevScaledInput=0  ExternalReset=none  TrackingMode=off  Kt=1  LimitOutput=off  UpperSaturationLimit=0.001  LowerSaturationLimit=-0.001  LinearizeAsGain=on  AntiWindupMode=none  Kb=1  POutMin=[]  POutMax=[]  IOutMin=[]  IOutMax=[]  DOutMin=[]  DOutMax=[]  NOutMin=[]  NOutMax=[]  SumOutMin=[]  SumOutMax=[]  SaturationOutMin=[]  SaturationOutMax=[]  PParamMin=[]  PParamMax=[]  IParamMin=[]  IParamMax=[]  DParamMin=[]  DParamMax=[]  NParamMin=[]  NParamMax=[]  KbParamMin=[]  KbParamMax=[]  KtParamMin=[]  KtParamMax=[]  KbOutMin=[]  KbOutMax=[]  KtOutMin=[]  KtOutMax=[]  IntegratorOutMin=[]  IntegratorOutMax=[]  FilterOutMin=[]  FilterOutMax=[]  SumI1OutMin=[]  SumI1OutMax=[]  SumI2OutMin=[]  SumI2OutMax=[]  SumI3OutMin=[]  SumI3OutMax=[]  SumI4OutMin=[]  SumI4OutMax=[]  SumDOutMin=[]  SumDOutMax=[]  DifferentiatorOutMin=[]  DifferentiatorOutMax=[]  FilterDiffOutCoefMin=[]  FilterDiffOutCoefMax=[]  ReciprocalOutMin=[]  ReciprocalOutMax=[]  SumDenOutMin=[]  SumDenOutMax=[]  SumNumOutMin=[]  SumNumOutMax=[]  DivideOutMin=[]  DivideOutMax=[]  IntegratorContinuousStateAttributes=''  IntegratorStateMustResolveToSignalObject=off  IntegratorRTWStateStorageClass=Auto  FilterContinuousStateAttributes=''  FilterStateMustResolveToSignalObject=off  FilterRTWStateStorageClass=Auto  ParallelPVariant=InternalParameters  IdealPVariant=Disabled  IVariant=InternalParameters  DVariant=Disabled  IntegratorVariant=Discrete  SatVariant=Disabled  AWVariant=Passthrough  PCopyVariant=Disabled  TRVariant=Disabled  FdbkBlocksVariant=Forward  IdealPFdbkVariant=Disabled  SatFdbkVariant=Disabled  DerivativeFilterVariant=Disabled  NVariant=Disabled  NCopyVariant=Disabled_SignalSpec  FilterICVariant=Disabled  IntegratorICVariant=InternalICs  ExternalResetVariant=Disabled  TRSumVariant=Passthrough  SumFdbkVariant=Disabled  SumVariant=Sum_PI
  PID Controller5 : simulink/Continuous/PID Controller  Controller=PI  Form=Parallel  TimeDomain=Discrete-time  SampleTime=ts  IntegratorMethod=Forward Euler  FilterMethod=Forward Euler  ControllerParametersSource=internal  P=0.00225  I=0.015  D=0  UseFilter=on  N=0  TunerSelectOption=Transfer Function Based (PID Tuner App)  InitialConditionSource=internal  InitialConditionForIntegrator=0  InitialConditionForFilter=0  DifferentiatorICPrevScaledInput=0  ExternalReset=none  TrackingMode=off  Kt=1  LimitOutput=off  UpperSaturationLimit=0.001  LowerSaturationLimit=-0.001  LinearizeAsGain=on  AntiWindupMode=none  Kb=1  POutMin=[]  POutMax=[]  IOutMin=[]  IOutMax=[]  DOutMin=[]  DOutMax=[]  NOutMin=[]  NOutMax=[]  SumOutMin=[]  SumOutMax=[]  SaturationOutMin=[]  SaturationOutMax=[]  PParamMin=[]  PParamMax=[]  IParamMin=[]  IParamMax=[]  DParamMin=[]  DParamMax=[]  NParamMin=[]  NParamMax=[]  KbParamMin=[]  KbParamMax=[]  KtParamMin=[]  KtParamMax=[]  KbOutMin=[]  KbOutMax=[]  KtOutMin=[]  KtOutMax=[]  IntegratorOutMin=[]  IntegratorOutMax=[]  FilterOutMin=[]  FilterOutMax=[]  SumI1OutMin=[]  SumI1OutMax=[]  SumI2OutMin=[]  SumI2OutMax=[]  SumI3OutMin=[]  SumI3OutMax=[]  SumI4OutMin=[]  SumI4OutMax=[]  SumDOutMin=[]  SumDOutMax=[]  DifferentiatorOutMin=[]  DifferentiatorOutMax=[]  FilterDiffOutCoefMin=[]  FilterDiffOutCoefMax=[]  ReciprocalOutMin=[]  ReciprocalOutMax=[]  SumDenOutMin=[]  SumDenOutMax=[]  SumNumOutMin=[]  SumNumOutMax=[]  DivideOutMin=[]  DivideOutMax=[]  IntegratorContinuousStateAttributes=''  IntegratorStateMustResolveToSignalObject=off  IntegratorRTWStateStorageClass=Auto  FilterContinuousStateAttributes=''  FilterStateMustResolveToSignalObject=off  FilterRTWStateStorageClass=Auto  ParallelPVariant=InternalParameters  IdealPVariant=Disabled  IVariant=InternalParameters  DVariant=Disabled  IntegratorVariant=Discrete  SatVariant=Disabled  AWVariant=Passthrough  PCopyVariant=Disabled  TRVariant=Disabled  FdbkBlocksVariant=Forward  IdealPFdbkVariant=Disabled  SatFdbkVariant=Disabled  DerivativeFilterVariant=Disabled  NVariant=Disabled  NCopyVariant=Disabled_SignalSpec  FilterICVariant=Disabled  IntegratorICVariant=InternalICs  ExternalResetVariant=Disabled  TRSumVariant=Passthrough  SumFdbkVariant=Disabled  SumVariant=Sum_PI
  filter{,1..5} (6 alike) : controlLibrary/filter  tc=1e-2  sampleTime=ts
  tRef : Outport  OutDataTypeStr=Bus: jointTorqueBus  Unit=N*m
  wires:
  Gain13/1 -> [RFA_w]
  Gain4/1 -> [UA_w]
  Bus Selector1/6 -> Gain16/1  "<leftFingerJointVel>"
  Bus Selector/2 -> Gain3/1  "<foreArmJointVel>"
  [FA_tRef] -> Bus Creator2/2  "FAtRef"
  Gain10/1 -> [GA_w]
  [GA_tRef] -> Bus Creator2/4  "GAtRef"
  Bus Selector1/1 -> Gain4/1  "<upperArmJointVel>"
  Bus Selector/1 -> Gain2/1  "<upperArmJointVel>"
  Gain7/1 -> [WA_w]
  w/1 -> Bus Selector1/1
  Bus Selector/3 -> Gain6/1  "<wristJointVel>"
  Bus Selector1/3 -> Gain7/1  "<wristJointVel>"
  Bus Selector1/2 -> Gain5/1  "<foreArmJointVel>"
  wRef/1 -> Bus Selector/1
  Gain6/1 -> [WA_wRef]
  Gain15/1 -> [LFA_wRef]
  Gain5/1 -> [FA_w]
  Bus Selector/4 -> Gain9/1  "<gripperJointVel>"
  [WA_tRef] -> Bus Creator2/3  "WAtRef"
  Gain9/1 -> [GA_wRef]
  Gain16/1 -> [LFA_w]
  Gain12/1 -> [RFA_wRef]
  Bus Selector1/5 -> Gain13/1  "<rightFingerJointVel>"
  Bus Selector/6 -> Gain15/1  "<leftFingerJointVel>"
  Gain3/1 -> [FA_wRef]
  [RFA_tRef] -> Bus Creator2/5  "RFAtRef"
  Bus Selector/5 -> Gain12/1  "<rightFingerJointVel>"
  Bus Selector1/4 -> Gain10/1  "<gripperJointVel>"
  Gain2/1 -> [UA_wRef]
  [LFA_tRef] -> Bus Creator2/6  "LFAtRef"
  [UA_tRef] -> Bus Creator2/1  "UAtRef"
  Bus Creator2/1 -> tRef/1  "torqueReference"
  [GA_w] -> filter3/2
  [RFA_wRef] -> filter4/1
  [FA_w] -> filter1/2
  [WA_wRef] -> filter2/1
  PID Controller2/1 -> [WA_tRef]
  PID Controller5/1 -> [LFA_tRef]
  [LFA_wRef] -> filter5/1
  PID Controller3/1 -> [GA_tRef]
  [FA_wRef] -> filter1/1
  PID Controller4/1 -> [RFA_tRef]
  [LFA_w] -> filter5/2
  [GA_wRef] -> filter3/1
  [RFA_w] -> filter4/2
  [UA_w] -> filter/2
  [UA_wRef] -> filter/1
  [WA_w] -> filter2/2
  PID Controller/1 -> [UA_tRef]
  filter/1 -> PID Controller/1
  filter1/1 -> PID Controller1/1
  PID Controller1/1 -> [FA_tRef]
  filter2/1 -> PID Controller2/1
  filter3/1 -> PID Controller3/1
  filter4/1 -> PID Controller4/1
  filter5/1 -> PID Controller5/1

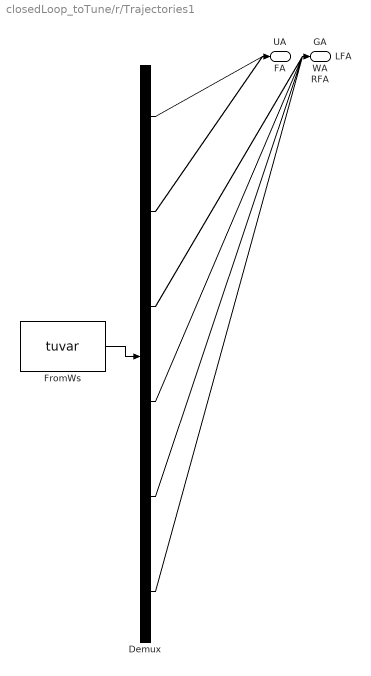
== system closedLoop_toTune/r/Trajectories1 ==
  Demux : Demux  Tag=STV Demux  Outputs=6
  FromWs : FromWorkspace  Tag=STV FromWs  VariableName=tuvar  SampleTime=0
      SigBuilderData=|
      | common.afterFinalStr = 'Extrapolate'
      | common.sampleTime = '0'
      | dataSet.timeRange = [0 20]
      | dataSet.name = 'jointMotion'
      | sbobj.Groups.Name = 'jointMotion'
      | sbobj.Groups.Signals(1).Name = 'UA'
      | sbobj.Groups.Signals(1).XData = [0 2.5 7.5 12.5 17.5 20]
      | sbobj.Groups.Signals(1).YData = [0 -90 -90 90 90 0]
      | sbobj.Groups.Signals(2).Name = 'FA'
      | sbobj.Groups.Signals(2).XData = [0 2.5 7.5 12.5 17.5 20]
      | sbobj.Groups.Signals(2).YData = [0 -45 -45 30 30 0]
      | sbobj.Groups.Signals(3).Name = 'WA'
      | sbobj.Groups.Signals(3).XData = [0 2.5 4.5 5.5 7.5 12.5 14.5 15.5 17.5 20]
      | sbobj.Groups.Signals(3).YData = [0 0 -90 -90 0 0 -90 -90 0 0]
      | sbobj.Groups.Signals(4).Name = 'GA'
      | sbobj.Groups.Signals(4).XData = [0 2.5 4.5 5.5 7.5 12.5 14.5 15.5 17.5 20]
      | sbobj.Groups.Signals(4).YData = [0 0 45 45 0 0 -45 -45 0 0]
      | sbobj.Groups.Signals(5).Name = 'RFA'
      | sbobj.Groups.Signals(5).XData = [0 4 4.5 5.5 6 14.5 15.5 20]
      | sbobj.Groups.Signals(5).YData = [136 136 136 150 150 150 136 136]
      | sbobj.Groups.Signals(6).Name = 'LFA'
      | sbobj.Groups.Signals(6).XData = [0 4 4.5 5.5 6 14.5 15.5 20]
      | sbobj.Groups.Signals(6).YData = [-136 -136 -136 -150 -150 -150 -136 -136]
      | sbobj.Groups.TimeRange = [0 20]
  UA : Outport  Tag=STV Outport
  FA : Outport  Tag=STV Outport  Port=2
  WA : Outport  Tag=STV Outport  Port=3
  GA : Outport  Tag=STV Outport  Port=4
  RFA : Outport  Tag=STV Outport  Port=5
  LFA : Outport  Tag=STV Outport  Port=6
  wires:
  FromWs/1 -> Demux/1
  Demux/1 -> UA/1
  Demux/2 -> FA/1
  Demux/3 -> WA/1
  Demux/4 -> GA/1
  Demux/5 -> RFA/1
  Demux/6 -> LFA/1
